simulink model "Thesis_MMC_WF_Modify"  (R2023a)
settings: Solver=VariableStepAuto  StartTime=0.0  StopTime=16  RelTol=1e-3
InitFcn:
  | % TS %
  | Ts_Control=4e-05;
  | Ts_Power=2e-05;
  | %% Main Circuit %%
  | % AC Line %
  | Vnom_Sec=333000;
  | Vnom_Pri=400000;
  | Pnom=1.0e+09;
  | Fnom=60;
  | Psc=2.0e+10;
  | P_Ld1=2/3*1e+09;
  | R_Startup=400;
  | Rxfo=0.003;
  | Lxfo=0.12;
  | P_Ld2=500e+03;
  | % MMC Parameter %
  | Larm_pu=0.15;
  | Rarm_pu=Larm_pu/100;
  | Zbase= Vnom_Sec^2/Pnom;
  | Larm=Larm_pu*(Zbase/(2*pi*Fnom));
  | Rarm=Rarm_pu*Zbase;
  | C_PM=1.758e-3;
  | w=2*pi*Fnom;
  | wc2=(2*w)^2;
  | Cfilter=1/(Larm*wc2);
  | Rfilter=1/(Cfilter*w)*30;
  | Topen_Filter=1e6;
  | K_V_dc=600000;
  | n=36;
  | Rg=100;
  | Cg=5e-08;
  | % HVDC Parameter %
  | R_cable=0.5;
  | L_cable=0.015;
  | %% Controller Parameter %%
  | % PLL %
  | Fn_filter=1000;
  | Zeta_filter=1;
  | % Active Power Regulator %
  | Kp_Preg=1/6;
  | Ki_Preg=1;
  | Limits_Preg=[0.8 1.2];
  | set_param('Thesis_MMC_WF_Modify/Controller/Active Power Regulator/Sum1','SampleTime','Ts_Control')
  | set_param('Thesis_MMC_WF_Modify/Controller/Active Power Regulator/Saturation','SampleTime','Ts_Control')
  | % Reactive Power Regulator %
  | Kp_Qreg=1/6;
  | Ki_Qreg=1;
  | Limits_Qreg=[-0.25 0.25];
  | set_param('Thesis_MMC_WF_Modify/Controller/Reactive Power Regulartor/Sum1','SampleTime','Ts_Control')
  | % Discrete Mean %
  | K1=3.2312e-30;
  | K2=-1.1369e-16;
  | Delay=0.02;
  | Vint=0;
  | Delay1=0.02004;
  | % DC Voltage Regulator %
  | Kp_VDCreg=4;
  | Ki_VDCreg=100;
  | Limits_VDCreg=[-2 2];
  | set_param('Thesis_MMC_WF_Modify/Controller/DC Voltage Regulator/Sum1','SampleTime','Ts_Control')
  | set_param('Thesis_MMC_WF_Modify/Controller/DC Voltage Regulator/Saturation','SampleTime','Ts_Control')
  | % Current Regulator %
  | Limits_Ireg=[-2 2];
  | Lff=0.075;
  | Rff=0.00075;
  | % PI Regulator %
  | Kp=0.6;
  | Ki=6;
  | UpperLimit=2;
  | LowerLimit=-2;
  | set_param('Thesis_MMC_WF_Modify/Controller/Current Regular/PI Regulator1/Sum1','SampleTime','Ts_Control')
  | set_param('Thesis_MMC_WF_Modify/Controller/Current Regular/PI Regulator1/Sum2','SampleTime','Ts_Control')
  | set_param('Thesis_MMC_WF_Modify/Controller/Current Regular/PI Regulator1/Gain1','SampleTime','Ts_Control')
  | set_param('Thesis_MMC_WF_Modify/Controller/Current Regular/PI Regulator1/Gain2','SampleTime','Ts_Control')
  | set_param('Thesis_MMC_WF_Modify/Controller/Current Regular/PI Regulator1/Saturation','SampleTime','Ts_Control')
  | set_param('Thesis_MMC_WF_Modify/Controller/Current Regular/PI Regulator2/Sum1','SampleTime','Ts_Control')
  | set_param('Thesis_MMC_WF_Modify/Controller/Current Regular/PI Regulator2/Sum2','SampleTime','Ts_Control')
  | set_param('Thesis_MMC_WF_Modify/Controller/Current Regular/PI Regulator2/Gain1','SampleTime','Ts_Control')
  | set_param('Thesis_MMC_WF_Modify/Controller/Current Regular/PI Regulator2/Gain2','SampleTime','Ts_Control')
  | set_param('Thesis_MMC_WF_Modify/Controller/Current Regular/PI Regulator2/Saturation','SampleTime','Ts_Control')
  | % PWM Generator %
  | pp=0;
  | for p=1:2:72
  | pp=pp+1;
  | SelectPulses1(p)=pp;
  | SelectPulses1(p+1)=pp+36;
  | end
  | Offse_Cr=0:0.000137377733816902958333333:35*0.000137377733816902958333333;
  | Fc=Fnom*3.37;
  | Tc=0.004945598417408506583333333;
  | %% Sequence & Slope %%
  | TBrk1_On=0.1;
  | TBrk2_On=1;
  | Ton_VDCreg=1.5;
  | Slope_Vdc_ref=128000;
  | Tramping_Vdc_ref=2;
  | Slope_Pref=0.5;
  | Ton_PQreg=4;
  | Tramping_Pref=4.2;
  | Slope_Qref=0.5;
  | Tramping_Qref=7.0;
  | Limits_Qreg=[-0.25 0.25];
  | %% Fault Time %%
  | T_Fault=10;
  | %% 12-Pulse %%
  | R_12_arm=0.001;
undefined symbols (not defined in the file): D1, Delta, Delta1, DiscIntNeverNeededParam, Lagging, Vnom_dc
libraries: spsSeriesRLCBranchLib x54, spsIGBTLib x24, spsBreakerLib x13, spsVoltageMeasurementLib x11, spsThreePhaseBreakerLib x11, spsThreePhaseVIMeasurementLib x9, spsIdealSwitchLib x8, simulink x7, spsDiscreteVariableTimeDelayLib x7, spsCurrentMeasurementLib x6, spsGroundLib x6, spsSecondOrderFilterLib x6
(part 1 of 3)
settings Model: SimulationMode=accelerator  Creator=GW Smart Grid Lab  LastModifiedBy=hwang22
settings OptimizationCC: ReuseModelBlockBuffer=off

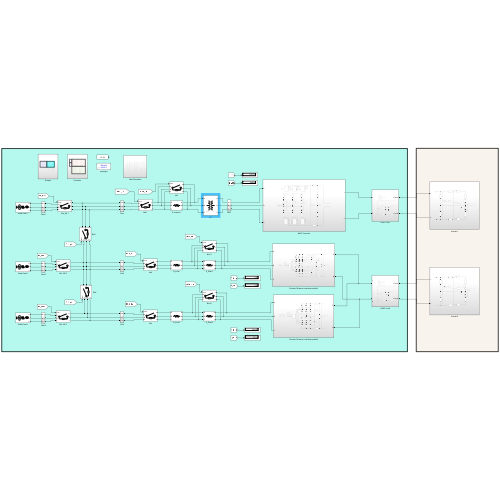
[thumbnail: Simulink's stored preview of the top-level diagram]
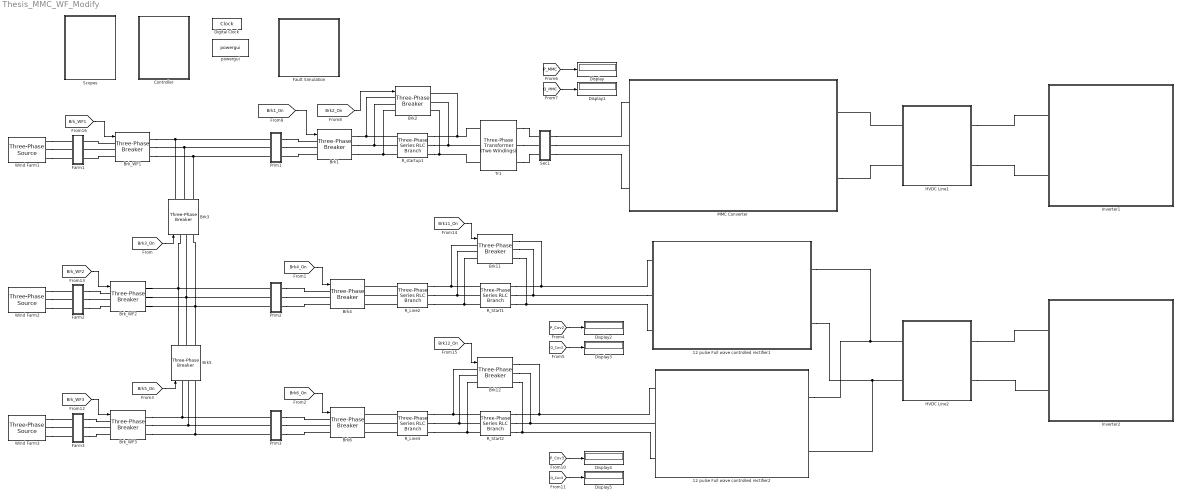
== system Thesis_MMC_WF_Modify ==
  12 pulse Full wave controlled rectifier1 : Subsystem
  12 pulse Full wave controlled rectifier2 : Subsystem
  Brk1 : spsThreePhaseBreakerLib/Three-Phase Breaker  InitialState=open  SwitchA=on  SwitchB=on  SwitchC=on  SwitchTimes=0.1  External=on  BreakerResistance=0.001  SnubberResistance=1e6  SnubberCapacitance=inf  Measurements=None
  Brk{3..6,11..12} (6 alike) : spsThreePhaseBreakerLib/Three-Phase Breaker  InitialState=open  SwitchA=on  SwitchB=on  SwitchC=on  SwitchTimes="[1/60  5/60]"  External=on  BreakerResistance=0.01  SnubberResistance=1e6  SnubberCapacitance=inf  Measurements=None
  Brk2 : spsThreePhaseBreakerLib/Three-Phase Breaker  InitialState=open  SwitchA=on  SwitchB=on  SwitchC=on  SwitchTimes=[30/60]*10000  External=on  BreakerResistance=0.01  SnubberResistance=1e6  SnubberCapacitance=inf  Measurements=None
  Brk_WF1 : spsThreePhaseBreakerLib/Three-Phase Breaker  InitialState=open  SwitchA=on  SwitchB=on  SwitchC=on  SwitchTimes="[1/60  5/60]"  External=on  BreakerResistance=0.01  SnubberResistance=1e6  SnubberCapacitance=inf  Measurements=None
  Brk_WF2 : spsThreePhaseBreakerLib/Three-Phase Breaker  InitialState=open  SwitchA=on  SwitchB=on  SwitchC=on  SwitchTimes="[1/60  5/60]"  External=on  BreakerResistance=0.01  SnubberResistance=1e6  SnubberCapacitance=inf  Measurements=None
  Brk_WF3 : spsThreePhaseBreakerLib/Three-Phase Breaker  InitialState=open  SwitchA=on  SwitchB=on  SwitchC=on  SwitchTimes="[1/60  5/60]"  External=on  BreakerResistance=0.01  SnubberResistance=1e6  SnubberCapacitance=inf  Measurements=None
  Controller : Subsystem
  Digital Clock : DigitalClock  SampleTime=Ts_Control
  Display{,1..5} (6 alike) : Display
      settings: Format=bank  Decimation=500
  Farm1 : Subsystem
  Farm2 : Subsystem
  Farm3 : Subsystem
  Fault Simulation : Subsystem
  HVDC Line1 : Subsystem
  HVDC Line2 : Subsystem
  Inverter1 : Subsystem
  Inverter2 : Subsystem
  MMC Converter : Subsystem
  Prim1 : Subsystem
  Prim2 : Subsystem
  Prim3 : Subsystem
  R_Line2 : spsThreePhaseSeriesRLCBranchLib/Three-Phase Series RLC Branch  LConnTagsString=A|B|C  RConnTagsString=A|B|C  BranchType=R  Resistance=10*0.007  Inductance=1e-3  Capacitance=1e-6  Measurements=None
  R_Line3 : spsThreePhaseSeriesRLCBranchLib/Three-Phase Series RLC Branch  LConnTagsString=A|B|C  RConnTagsString=A|B|C  BranchType=R  Resistance=10*0.007  Inductance=1e-3  Capacitance=1e-6  Measurements=None
  R_Start1 : spsThreePhaseSeriesRLCBranchLib/Three-Phase Series RLC Branch  LConnTagsString=A|B|C  RConnTagsString=A|B|C  BranchType=R  Resistance=540*0.01  Inductance=1e-3  Capacitance=1e-6  Measurements=None
  R_Start2 : spsThreePhaseSeriesRLCBranchLib/Three-Phase Series RLC Branch  LConnTagsString=A|B|C  RConnTagsString=A|B|C  BranchType=R  Resistance=540*0.01  Inductance=1e-3  Capacitance=1e-6  Measurements=None
  R_startup1 : spsThreePhaseSeriesRLCBranchLib/Three-Phase Series RLC Branch  LConnTagsString=A|B|C  RConnTagsString=A|B|C  BranchType=R  Resistance=R_Startup/100  Inductance=1e-3  Capacitance=1e-6  Measurements=None
  Scopes : Subsystem
  Sec1 : Subsystem
  Tr1 : spsThreePhaseTransformerTwoWindingsLib/Three-Phase Transformer (Two Windings)  Winding1Connection=Yg  Winding2Connection=Y  CoreType=Three single-phase transformers  SetSaturation=off  Hysteresis=off  DataFile='hysteresis'  SetInitialFlux=off  Measurements=None  UNITS=pu  NominalPower=[ Pnom , Fnom ]  Winding1="[ Vnom_Pri*0.1 , Rxfo/2,  Lxfo/2 ]"  Winding2="[ Vnom_Sec , Rxfo/2,  Lxfo/2 ]"  Rm=1000  Lm=1000  L0=0.5  Saturation=[ 0,0 ; 0.0024,1.2 ; 1.0,1.52 ]  InitialFluxes=[ 0.8 , -0.8 , 0.7 ]  BreakLoop=off  DiscreteSolver=Trapezoidal iterative  DataType=off  TransfoNumber=1
  Wind Farm1 : spsThreePhaseSourceLib/Three-Phase Source  InternalConnection=Yg  VoltagePhases=off  Voltage=Vnom_Pri*0.099  PhaseAngle=0  Voltage_phases=[25e3 25e3 25e3]/sqrt(3)  PhaseAngles_phases=[0 -120 +120]  Frequency=Fnom  NonIdealSource=on  SpecifyImpedance=on  Resistance=0.8929  Inductance=16.58e-3  ShortCircuitLevel=Psc  BaseVoltage=Vnom_Pri*0.1  XRratio=7  BusType=PQ  Pref=1.0e9  Qref=2.5e8  Prefabc=[10e3, 10e3, 10e3]  Qrefabc=[0, 0, 0]  Qmin=-inf  Qmax=inf
  Wind Farm2 : spsThreePhaseSourceLib/Three-Phase Source  InternalConnection=Yg  VoltagePhases=off  Voltage=Vnom_Pri*0.099  PhaseAngle=0  Voltage_phases=[25e3 25e3 25e3]/sqrt(3)  PhaseAngles_phases=[0 -120 +120]  Frequency=Fnom  NonIdealSource=on  SpecifyImpedance=on  Resistance=0.8929  Inductance=16.58e-3  ShortCircuitLevel=Psc  BaseVoltage=Vnom_Pri*0.1  XRratio=7  BusType=PQ  Pref=1.2e9  Qref=2.5e8  Prefabc=[10e3, 10e3, 10e3]  Qrefabc=[0, 0, 0]  Qmin=-inf  Qmax=inf
  Wind Farm3 : spsThreePhaseSourceLib/Three-Phase Source  InternalConnection=Yg  VoltagePhases=off  Voltage=Vnom_Pri*0.099  PhaseAngle=0  Voltage_phases=[25e3 25e3 25e3]/sqrt(3)  PhaseAngles_phases=[0 -120 +120]  Frequency=Fnom  NonIdealSource=on  SpecifyImpedance=on  Resistance=0.8929  Inductance=16.58e-3  ShortCircuitLevel=Psc  BaseVoltage=Vnom_Pri*0.1  XRratio=7  BusType=PQ  Pref=1.0e9  Qref=2.5e8  Prefabc=[10e3, 10e3, 10e3]  Qrefabc=[0, 0, 0]  Qmin=-inf  Qmax=inf
  powergui : spspowerguiLib/powergui  Priority=1  SimulationMode=Discrete  SampleTime=Ts_Power  frequency=60  Iterations=50  frequencyindice=60  Pbase=100e6  ErrMax=1e-4  UnitsV=kV  UnitsW=MW  buscounter=0  FunctionMessages=off  echomessages=off  EnableUseOfTLC=off  CurrentSourceSwitches=off  DisableSnubberDevices=off  DisableRonSwitches=off  DisableVfSwitches=off  DisplayEquations=off  AutomaticDiscreteSolvers=off  SolverType=Tustin/Backward Euler (TBE)  Interpol=off  ExternalGateDelay=off  methode=off  Ts=100  x0status=blocks  SPID=on  SwTol=0  HookPort=off  NonlinearTolerance=1e-4  nMaxIteration=100  ContinueOnMaxIteration=off  RestoreLinks=warning  ResistiveCurrentMeasurement=off  Frange=[0:2:500]  Ylog=off  Xlog=on  ShowGrid=off  save=off  variable=ZData  structure=0  ZoomFFT=off  StartTime=0.0  cycles=1  DisplayStyle=1  fundamental=60  FreqAxis=off  MaxFrequency=1000  frequencyindicesteady=1  RmsSteady=1  display=off
  wires:
  [Brk2_On] -> Brk2/1
  [Brk1_On] -> Brk1/1
  [Brk3_On] -> Brk3/1
  [Brk4_On] -> Brk4/1
  [Brk6_On] -> Brk6/1
  [Brk5_On] -> Brk5/1
  [P_MMC] -> Display/1
  [Q_MMC] -> Display1/1
  [Brk11_On] -> Brk11/1
  [Brk12_On] -> Brk12/1
  [Q_Cov2] -> Display3/1
  [P_Cov2] -> Display2/1
  [P_Cov3] -> Display4/1
  [Q_Cov3] -> Display5/1
  [Brk_WF3] -> Brk_WF3/1
  [Brk_WF2] -> Brk_WF2/1
  [Brk_WF1] -> Brk_WF1/1
  connections:
  R_startup1/RConn1 -- Tr1/LConn1 -- Brk2/RConn1
  Tr1/RConn3 -- Sec1/LConn3
  Tr1/RConn2 -- Sec1/LConn2
  Brk2/LConn1 -- Brk1/RConn1 -- R_startup1/LConn1
  Brk2/LConn2 -- Brk1/RConn2 -- R_startup1/LConn2
  Brk2/LConn3 -- Brk1/RConn3 -- R_startup1/LConn3
  Tr1/RConn1 -- Sec1/LConn1
  R_startup1/RConn2 -- Tr1/LConn2 -- Brk2/RConn2
  R_startup1/RConn3 -- Tr1/LConn3 -- Brk2/RConn3
  HVDC Line1/RConn1 -- Inverter1/LConn1
  HVDC Line1/RConn2 -- Inverter1/LConn2
  Brk1/LConn3 -- Prim1/RConn3
  Prim1/RConn2 -- Brk1/LConn2
  Prim1/RConn1 -- Brk1/LConn1
  Sec1/RConn1 -- MMC Converter/LConn1
  Sec1/RConn2 -- MMC Converter/LConn2
  Sec1/RConn3 -- MMC Converter/LConn3
  Brk5/RConn2 -- Brk_WF2/RConn2 -- Prim2/LConn2 -- Brk3/LConn2
  Brk5/RConn1 -- Brk_WF2/RConn1 -- Brk3/LConn1 -- Prim2/LConn1
  12 pulse Full wave controlled rectifier1/LConn1 -- R_Start1/RConn1 -- Brk11/RConn1
  12 pulse Full wave controlled rectifier1/LConn2 -- R_Start1/RConn2 -- Brk11/RConn2
  12 pulse Full wave controlled rectifier1/LConn3 -- R_Start1/RConn3 -- Brk11/RConn3
  HVDC Line1/LConn1 -- MMC Converter/RConn1
  MMC Converter/RConn2 -- HVDC Line1/LConn2
  12 pulse Full wave controlled rectifier2/LConn1 -- Brk12/RConn1 -- R_Start2/RConn1
  R_Start2/LConn2 -- R_Line3/RConn2 -- Brk12/LConn2
  R_Start2/LConn3 -- R_Line3/RConn3 -- Brk12/LConn3
  12 pulse Full wave controlled rectifier1/RConn1 -- 12 pulse Full wave controlled rectifier2/RConn1 -- HVDC Line2/LConn1
  Prim2/RConn3 -- Brk4/LConn3
  Prim2/RConn2 -- Brk4/LConn2
  Prim2/RConn1 -- Brk4/LConn1
  Prim3/RConn1 -- Brk6/LConn1
  Prim3/RConn2 -- Brk6/LConn2
  Prim3/RConn3 -- Brk6/LConn3
  HVDC Line2/RConn1 -- Inverter2/LConn1
  HVDC Line2/RConn2 -- Inverter2/LConn2
  Prim3/LConn1 -- Brk5/LConn1 -- Brk_WF3/RConn1
  HVDC Line2/LConn2 -- 12 pulse Full wave controlled rectifier1/RConn2 -- 12 pulse Full wave controlled rectifier2/RConn2
  Wind Farm1/RConn1 -- Farm1/LConn1
  Wind Farm1/RConn2 -- Farm1/LConn2
  Wind Farm1/RConn3 -- Farm1/LConn3
  R_Start1/LConn1 -- R_Line2/RConn1 -- Brk11/LConn1
  R_Start1/LConn2 -- R_Line2/RConn2 -- Brk11/LConn2
  R_Start1/LConn3 -- R_Line2/RConn3 -- Brk11/LConn3
  Brk12/RConn3 -- R_Start2/RConn3 -- 12 pulse Full wave controlled rectifier2/LConn3
  R_Start2/LConn1 -- R_Line3/RConn1 -- Brk12/LConn1
  Brk12/RConn2 -- R_Start2/RConn2 -- 12 pulse Full wave controlled rectifier2/LConn2
  Wind Farm2/RConn1 -- Farm2/LConn1
  Wind Farm2/RConn2 -- Farm2/LConn2
  Wind Farm2/RConn3 -- Farm2/LConn3
  Wind Farm3/RConn1 -- Farm3/LConn1
  Wind Farm3/RConn2 -- Farm3/LConn2
  Wind Farm3/RConn3 -- Farm3/LConn3
  Prim3/LConn3 -- Brk_WF3/RConn3 -- Brk5/LConn3
  Prim3/LConn2 -- Brk_WF3/RConn2 -- Brk5/LConn2
  Brk5/RConn3 -- Brk_WF2/RConn3 -- Prim2/LConn3 -- Brk3/LConn3
  Brk_WF1/RConn1 -- Brk3/RConn1 -- Prim1/LConn1
  Brk_WF1/RConn2 -- Brk3/RConn2 -- Prim1/LConn2
  Brk_WF1/RConn3 -- Brk3/RConn3 -- Prim1/LConn3
  Brk_WF1/LConn1 -- Farm1/RConn1
  Brk_WF1/LConn2 -- Farm1/RConn2
  Brk_WF1/LConn3 -- Farm1/RConn3
  Farm2/RConn3 -- Brk_WF2/LConn3
  Farm2/RConn2 -- Brk_WF2/LConn2
  Farm2/RConn1 -- Brk_WF2/LConn1
  Farm3/RConn3 -- Brk_WF3/LConn3
  Farm3/RConn2 -- Brk_WF3/LConn2
  Farm3/RConn1 -- Brk_WF3/LConn1
  R_Line2/LConn1 -- Brk4/RConn1
  R_Line2/LConn2 -- Brk4/RConn2
  R_Line2/LConn3 -- Brk4/RConn3
  R_Line3/LConn2 -- Brk6/RConn2
  R_Line3/LConn3 -- Brk6/RConn3
  R_Line3/LConn1 -- Brk6/RConn1

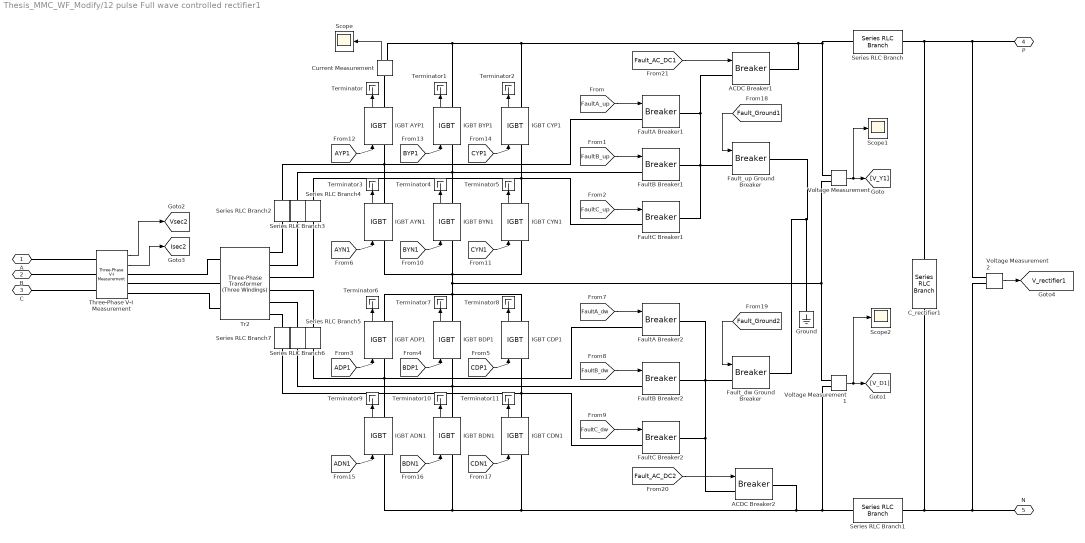
== system Thesis_MMC_WF_Modify/12 pulse Full wave controlled rectifier1 ==
  ACDC Breaker1 : spsBreakerLib/Breaker  InitialState=0  SwitchingTimes="[1/60  5/60]"  External=on  BreakerResistance=0.01  SnubberResistance=1e6  SnubberCapacitance=inf  Measurements=None  MoreParameters=on  NoBreakLoop=off
  ACDC Breaker2 : spsBreakerLib/Breaker  InitialState=0  SwitchingTimes="[1/60  5/60]"  External=on  BreakerResistance=0.01  SnubberResistance=1e6  SnubberCapacitance=inf  Measurements=None  MoreParameters=on  NoBreakLoop=off
  C_rectifier1 : spsSeriesRLCBranchLib/Series RLC Branch  LConnTagsString=__new0  RConnTagsString=__new0  BranchType=C  Resistance=1  Inductance=1e-3  SetiL0=off  InitialCurrent=0  Capacitance=5e-4  Setx0=off  InitialVoltage=0  Measurements=None
  Current Measurement : spsCurrentMeasurementLib/Current Measurement  PhasorSimulation=off  OutputType=Complex  PSBequivalent=0
  FaultA Breaker1 : spsBreakerLib/Breaker  InitialState=0  SwitchingTimes="[1/60  5/60]"  External=on  BreakerResistance=0.01  SnubberResistance=1e6  SnubberCapacitance=inf  Measurements=None  MoreParameters=on  NoBreakLoop=off
  FaultA Breaker2 : spsBreakerLib/Breaker  InitialState=0  SwitchingTimes="[1/60  5/60]"  External=on  BreakerResistance=0.01  SnubberResistance=1e6  SnubberCapacitance=inf  Measurements=None  MoreParameters=on  NoBreakLoop=off
  FaultB Breaker1 : spsBreakerLib/Breaker  InitialState=0  SwitchingTimes="[1/60  5/60]"  External=on  BreakerResistance=0.01  SnubberResistance=1e6  SnubberCapacitance=inf  Measurements=None  MoreParameters=on  NoBreakLoop=off
  FaultB Breaker2 : spsBreakerLib/Breaker  InitialState=0  SwitchingTimes="[1/60  5/60]"  External=on  BreakerResistance=0.01  SnubberResistance=1e6  SnubberCapacitance=inf  Measurements=None  MoreParameters=on  NoBreakLoop=off
  FaultC Breaker1 : spsBreakerLib/Breaker  InitialState=0  SwitchingTimes="[1/60  5/60]"  External=on  BreakerResistance=0.01  SnubberResistance=1e6  SnubberCapacitance=inf  Measurements=None  MoreParameters=on  NoBreakLoop=off
  FaultC Breaker2 : spsBreakerLib/Breaker  InitialState=0  SwitchingTimes="[1/60  5/60]"  External=on  BreakerResistance=0.01  SnubberResistance=1e6  SnubberCapacitance=inf  Measurements=None  MoreParameters=on  NoBreakLoop=off
  Fault_dw Ground Breaker : spsBreakerLib/Breaker  InitialState=0  SwitchingTimes="[1/60  5/60]"  External=on  BreakerResistance=0.01  SnubberResistance=1e6  SnubberCapacitance=inf  Measurements=None  MoreParameters=on  NoBreakLoop=off
  Fault_up Ground Breaker : spsBreakerLib/Breaker  InitialState=0  SwitchingTimes="[1/60  5/60]"  External=on  BreakerResistance=0.01  SnubberResistance=1e6  SnubberCapacitance=inf  Measurements=None  MoreParameters=on  NoBreakLoop=off
  Ground : spsGroundLib/Ground  LConnTagsString=a
  IGBT ADN1 : spsIGBTLib/IGBT  Ron=0.001  Lon=0  Vf=1  Tf=1e-6  Tt=2e-6  IC=0  Rs=1e5  Cs=inf  Measurements=on
  IGBT ADP1 : spsIGBTLib/IGBT  Ron=0.001  Lon=0  Vf=1  Tf=1e-6  Tt=2e-6  IC=0  Rs=1e5  Cs=inf  Measurements=on
  IGBT AYN1 : spsIGBTLib/IGBT  Ron=0.001  Lon=0  Vf=1  Tf=1e-6  Tt=2e-6  IC=0  Rs=1e5  Cs=inf  Measurements=on
  IGBT AYP1 : spsIGBTLib/IGBT  Ron=0.001  Lon=0  Vf=1  Tf=1e-6  Tt=2e-6  IC=0  Rs=1e5  Cs=inf  Measurements=on
  IGBT BDN1 : spsIGBTLib/IGBT  Ron=0.001  Lon=0  Vf=1  Tf=1e-6  Tt=2e-6  IC=0  Rs=1e5  Cs=inf  Measurements=on
  IGBT BDP1 : spsIGBTLib/IGBT  Ron=0.001  Lon=0  Vf=1  Tf=1e-6  Tt=2e-6  IC=0  Rs=1e5  Cs=inf  Measurements=on
  IGBT BYN1 : spsIGBTLib/IGBT  Ron=0.001  Lon=0  Vf=1  Tf=1e-6  Tt=2e-6  IC=0  Rs=1e5  Cs=inf  Measurements=on
  IGBT BYP1 : spsIGBTLib/IGBT  Ron=0.001  Lon=0  Vf=1  Tf=1e-6  Tt=2e-6  IC=0  Rs=1e5  Cs=inf  Measurements=on
  IGBT CDN1 : spsIGBTLib/IGBT  Ron=0.001  Lon=0  Vf=1  Tf=1e-6  Tt=2e-6  IC=0  Rs=1e5  Cs=inf  Measurements=on
  IGBT CDP1 : spsIGBTLib/IGBT  Ron=0.001  Lon=0  Vf=1  Tf=1e-6  Tt=2e-6  IC=0  Rs=1e5  Cs=inf  Measurements=on
  IGBT CYN1 : spsIGBTLib/IGBT  Ron=0.001  Lon=0  Vf=1  Tf=1e-6  Tt=2e-6  IC=0  Rs=1e5  Cs=inf  Measurements=on
  IGBT CYP1 : spsIGBTLib/IGBT  Ron=0.001  Lon=0  Vf=1  Tf=1e-6  Tt=2e-6  IC=0  Rs=1e5  Cs=inf  Measurements=on
  Scope : Scope
  Scope1 : Scope
  Scope2 : Scope
  Series RLC Branch : spsSeriesRLCBranchLib/Series RLC Branch  LConnTagsString=__new0  RConnTagsString=__new0  BranchType=L  Resistance=1  Inductance=0.0004  SetiL0=off  InitialCurrent=0  Capacitance=1e-6  Setx0=off  InitialVoltage=0  Measurements=None
  Series RLC Branch1 : spsSeriesRLCBranchLib/Series RLC Branch  LConnTagsString=__new0  RConnTagsString=__new0  BranchType=L  Resistance=1  Inductance=0.0004  SetiL0=off  InitialCurrent=0  Capacitance=1e-6  Setx0=off  InitialVoltage=0  Measurements=None
  Series RLC Branch{2..7} (6 alike) : spsSeriesRLCBranchLib/Series RLC Branch  LConnTagsString=__new0  RConnTagsString=__new0  BranchType=RL  Resistance=R_12_arm  Inductance=1e-3  SetiL0=off  InitialCurrent=0  Capacitance=1e-6  Setx0=off  InitialVoltage=0  Measurements=None
  Terminator{,1..11} (12 alike) : Terminator
  Three-Phase V-I Measurement : spsThreePhaseVIMeasurementLib/Three-Phase V-I Measurement  VoltageMeasurement=phase-to-ground  SetLabelV=off  LabelV=Vabc  Vpu=off  VpuLL=off  CurrentMeasurement=yes  SetLabelI=off  LabelI=Iabc  Ipu=off  Pbase=100e6  Vbase=500e3  OutputType=Complex  PhasorSimulation=off  PSBequivalent=0
  Tr2 : spsThreePhaseTransformerThreeWindingsLib/Three-Phase Transformer (Three Windings)  Winding1Connection=Yg  Winding2Connection=Y  Winding3Connection=Delta (D1)  CoreType=Three single-phase transformers  SetSaturation=off  Hysteresis=off  DataFile='hysteresis'  SetInitialFlux=off  Measurements=None  UNITS=pu  NominalPower=[ 2.5e9 , 60 ]  Winding1=[ 4e+5*0.1 , 0.002 , 0.08 ]  Winding2=[ 2.675e+5 , 0.002 , 0.08 ]  Winding3=[2.675e+5 , 0.002 , 0.08 ]  Rm=1000  Lm=1000  L0=0.5  Saturation=[ 0,0 ; 0.0024,1.2 ; 1.0,1.52 ]  InitialFluxes=[0.8 -0.8 0.7]  BreakLoop=off  DiscreteSolver=Trapezoidal iterative  DataType=off  TransfoNumber=1
      settings: LibrarySourceBlock=|
      | sps_lib/Power Grid Elements/Three-Phase
      | Transformer
      | (Three Windings)
  Voltage Measurement : spsVoltageMeasurementLib/Voltage Measurement  PhasorSimulation=off  OutputType=Complex  PSBequivalent=0
  Voltage Measurement1 : spsVoltageMeasurementLib/Voltage Measurement  PhasorSimulation=off  OutputType=Complex  PSBequivalent=0
  Voltage Measurement2 : spsVoltageMeasurementLib/Voltage Measurement  PhasorSimulation=off  OutputType=Complex  PSBequivalent=0
  A : PMIOPort  Side=Left
  B : PMIOPort  Port=2  Side=Left
  C : PMIOPort  Port=3  Side=Left
  P : PMIOPort  Port=4  Side=Right
  N : PMIOPort  Port=5  Side=Right
  tag scope: Isec2=global, V_rectifier1=global, Vsec2=global
  wires:
  IGBT BDN1/1 -> Terminator10/1
  IGBT CYP1/1 -> Terminator2/1
  IGBT BDP1/1 -> Terminator7/1
  IGBT AYN1/1 -> Terminator3/1
  IGBT BYP1/1 -> Terminator1/1
  [BYN1] -> IGBT BYN1/1
  IGBT CDN1/1 -> Terminator11/1
  [CYP1] -> IGBT CYP1/1
  IGBT CYN1/1 -> Terminator5/1
  IGBT AYP1/1 -> Terminator/1
  [BDN1] -> IGBT BDN1/1
  [BDP1] -> IGBT BDP1/1
  [CDN1] -> IGBT CDN1/1
  [BYP1] -> IGBT BYP1/1
  [CDP1] -> IGBT CDP1/1
  IGBT CDP1/1 -> Terminator8/1
  IGBT BYN1/1 -> Terminator4/1
  [ADP1] -> IGBT ADP1/1
  [ADN1] -> IGBT ADN1/1
  [AYN1] -> IGBT AYN1/1
  [CYN1] -> IGBT CYN1/1
  IGBT ADP1/1 -> Terminator6/1
  IGBT ADN1/1 -> Terminator9/1
  Voltage Measurement/1 -> Scope1/1, [V_Y1]
  Voltage Measurement1/1 -> Scope2/1, [V_D1]
  Three-Phase V-I Measurement/1 -> [Vsec2]
  Three-Phase V-I Measurement/2 -> [Isec2]
  Voltage Measurement2/1 -> [V_rectifier1]
  [FaultA_up] -> FaultA Breaker1/1
  [FaultB_up] -> FaultB Breaker1/1
  [FaultC_up] -> FaultC Breaker1/1
  [FaultA_dw] -> FaultA Breaker2/1
  [FaultB_dw] -> FaultB Breaker2/1
  [FaultC_dw] -> FaultC Breaker2/1
  [Fault_Ground1] -> Fault_up Ground Breaker/1
  [Fault_Ground2] -> Fault_dw Ground Breaker/1
  [Fault_AC_DC2] -> ACDC Breaker2/1
  [Fault_AC_DC1] -> ACDC Breaker1/1
  Current Measurement/1 -> Scope/1
  [AYP1] -> IGBT AYP1/1
  connections:
  IGBT ADN1/RConn1 -- Series RLC Branch5/RConn1 -- FaultA Breaker2/LConn1 -- IGBT ADP1/LConn1
  Voltage Measurement/LConn1 -- Series RLC Branch/LConn1 -- ACDC Breaker1/RConn1 -- IGBT CYP1/RConn1 -- Current Measurement/RConn1 -- IGBT BYP1/RConn1
  FaultA Breaker1/LConn1 -- Series RLC Branch2/LConn1 -- IGBT AYN1/RConn1 -- IGBT AYP1/LConn1
  IGBT CDP1/RConn1 -- Voltage Measurement1/LConn1 -- Voltage Measurement/LConn2 -- IGBT CYN1/LConn1 -- IGBT BYN1/LConn1 -- IGBT AYN1/LConn1 -- IGBT BDP1/RConn1 -- IGBT ADP1/RConn1
  IGBT CYN1/RConn1 -- Series RLC Branch4/LConn1 -- FaultC Breaker1/LConn1 -- IGBT CYP1/LConn1
  FaultA Breaker2/RConn1 -- FaultC Breaker2/RConn1 -- ACDC Breaker2/LConn1 -- Fault_dw Ground Breaker/LConn1 -- FaultB Breaker2/RConn1
  FaultB Breaker1/LConn1 -- IGBT BYP1/LConn1 -- Series RLC Branch3/LConn1 -- IGBT BYN1/RConn1
  IGBT CDN1/RConn1 -- Series RLC Branch7/RConn1 -- FaultC Breaker2/LConn1 -- IGBT CDP1/LConn1
  IGBT BDN1/RConn1 -- Series RLC Branch6/RConn1 -- IGBT BDP1/LConn1 -- FaultB Breaker2/LConn1
  Three-Phase V-I Measurement/RConn1 -- Tr2/LConn1
  Three-Phase V-I Measurement/RConn3 -- Tr2/LConn3
  Three-Phase V-I Measurement/RConn2 -- Tr2/LConn2
  A/RConn1 -- Three-Phase V-I Measurement/LConn1
  B/RConn1 -- Three-Phase V-I Measurement/LConn2
  C/RConn1 -- Three-Phase V-I Measurement/LConn3
  Voltage Measurement2/LConn1 -- C_rectifier1/LConn1 -- Series RLC Branch/RConn1 -- P/RConn1
  Voltage Measurement2/LConn2 -- Series RLC Branch1/RConn1 -- C_rectifier1/RConn1 -- N/RConn1
  Fault_up Ground Breaker/RConn1 -- Fault_dw Ground Breaker/RConn1 -- Ground/LConn1
  Voltage Measurement1/LConn2 -- Series RLC Branch1/LConn1 -- ACDC Breaker2/RConn1 -- IGBT CDN1/LConn1 -- IGBT BDN1/LConn1 -- IGBT ADN1/LConn1
  FaultA Breaker1/RConn1 -- Fault_up Ground Breaker/LConn1 -- FaultC Breaker1/RConn1 -- FaultB Breaker1/RConn1 -- ACDC Breaker1/LConn1
  Tr2/RConn1 -- Series RLC Branch2/RConn1
  Tr2/RConn2 -- Series RLC Branch3/RConn1
  Tr2/RConn3 -- Series RLC Branch4/RConn1
  Tr2/RConn4 -- Series RLC Branch5/LConn1
  Tr2/RConn5 -- Series RLC Branch6/LConn1
  Tr2/RConn6 -- Series RLC Branch7/LConn1
  IGBT AYP1/RConn1 -- Current Measurement/LConn1

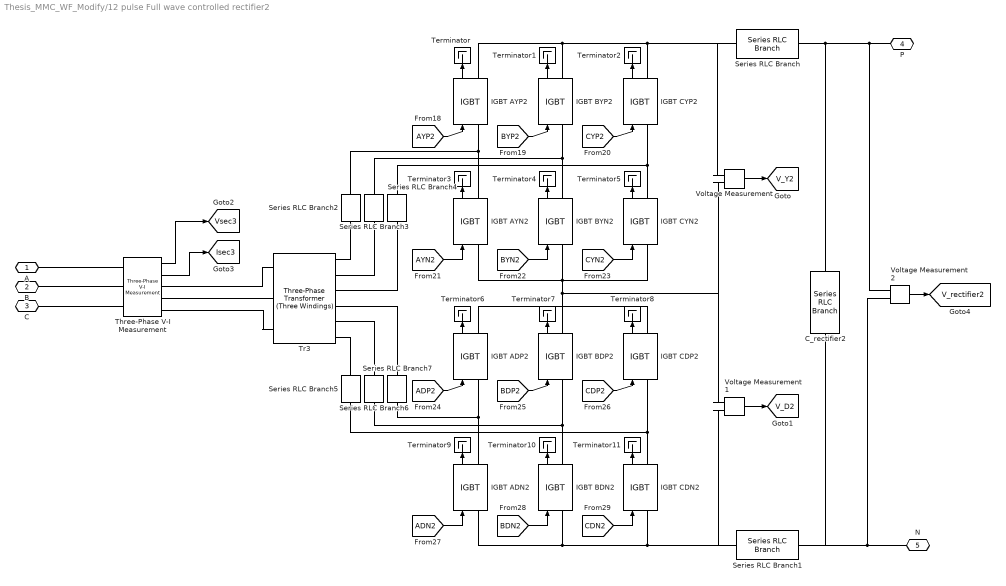
== system Thesis_MMC_WF_Modify/12 pulse Full wave controlled rectifier2 ==
  C_rectifier2 : spsSeriesRLCBranchLib/Series RLC Branch  LConnTagsString=__new0  RConnTagsString=__new0  BranchType=C  Resistance=1  Inductance=1e-3  SetiL0=off  InitialCurrent=0  Capacitance=5e-4  Setx0=off  InitialVoltage=0  Measurements=None
  IGBT ADN2 : spsIGBTLib/IGBT  Ron=0.001  Lon=0  Vf=1  Tf=1e-6  Tt=2e-6  IC=0  Rs=1e5  Cs=inf  Measurements=on
  IGBT ADP2 : spsIGBTLib/IGBT  Ron=0.001  Lon=0  Vf=1  Tf=1e-6  Tt=2e-6  IC=0  Rs=1e5  Cs=inf  Measurements=on
  IGBT AYN2 : spsIGBTLib/IGBT  Ron=0.001  Lon=0  Vf=1  Tf=1e-6  Tt=2e-6  IC=0  Rs=1e5  Cs=inf  Measurements=on
  IGBT AYP2 : spsIGBTLib/IGBT  Ron=0.001  Lon=0  Vf=1  Tf=1e-6  Tt=2e-6  IC=0  Rs=1e5  Cs=inf  Measurements=on
  IGBT BDN2 : spsIGBTLib/IGBT  Ron=0.001  Lon=0  Vf=1  Tf=1e-6  Tt=2e-6  IC=0  Rs=1e5  Cs=inf  Measurements=on
  IGBT BDP2 : spsIGBTLib/IGBT  Ron=0.001  Lon=0  Vf=1  Tf=1e-6  Tt=2e-6  IC=0  Rs=1e5  Cs=inf  Measurements=on
  IGBT BYN2 : spsIGBTLib/IGBT  Ron=0.001  Lon=0  Vf=1  Tf=1e-6  Tt=2e-6  IC=0  Rs=1e5  Cs=inf  Measurements=on
  IGBT BYP2 : spsIGBTLib/IGBT  Ron=0.001  Lon=0  Vf=1  Tf=1e-6  Tt=2e-6  IC=0  Rs=1e5  Cs=inf  Measurements=on
  IGBT CDN2 : spsIGBTLib/IGBT  Ron=0.001  Lon=0  Vf=1  Tf=1e-6  Tt=2e-6  IC=0  Rs=1e5  Cs=inf  Measurements=on
  IGBT CDP2 : spsIGBTLib/IGBT  Ron=0.001  Lon=0  Vf=1  Tf=1e-6  Tt=2e-6  IC=0  Rs=1e5  Cs=inf  Measurements=on
  IGBT CYN2 : spsIGBTLib/IGBT  Ron=0.001  Lon=0  Vf=1  Tf=1e-6  Tt=2e-6  IC=0  Rs=1e5  Cs=inf  Measurements=on
  IGBT CYP2 : spsIGBTLib/IGBT  Ron=0.001  Lon=0  Vf=1  Tf=1e-6  Tt=2e-6  IC=0  Rs=1e5  Cs=inf  Measurements=on
  Series RLC Branch : spsSeriesRLCBranchLib/Series RLC Branch  LConnTagsString=__new0  RConnTagsString=__new0  BranchType=L  Resistance=1  Inductance=0.0004  SetiL0=off  InitialCurrent=0  Capacitance=1e-6  Setx0=off  InitialVoltage=0  Measurements=None
  Series RLC Branch1 : spsSeriesRLCBranchLib/Series RLC Branch  LConnTagsString=__new0  RConnTagsString=__new0  BranchType=L  Resistance=1  Inductance=0.0004  SetiL0=off  InitialCurrent=0  Capacitance=1e-6  Setx0=off  InitialVoltage=0  Measurements=None
  Series RLC Branch{2..7} (6 alike) : spsSeriesRLCBranchLib/Series RLC Branch  LConnTagsString=__new0  RConnTagsString=__new0  BranchType=RL  Resistance=R_12_arm  Inductance=1e-3  SetiL0=off  InitialCurrent=0  Capacitance=1e-6  Setx0=off  InitialVoltage=0  Measurements=None
  Terminator{,1..11} (12 alike) : Terminator
  Three-Phase V-I Measurement : spsThreePhaseVIMeasurementLib/Three-Phase V-I Measurement  VoltageMeasurement=phase-to-ground  SetLabelV=off  LabelV=Vabc  Vpu=off  VpuLL=off  CurrentMeasurement=yes  SetLabelI=off  LabelI=Iabc  Ipu=off  Pbase=100e6  Vbase=500e3  OutputType=Complex  PhasorSimulation=off  PSBequivalent=0
  Tr3 : spsThreePhaseTransformerThreeWindingsLib/Three-Phase Transformer (Three Windings)  Winding1Connection=Yg  Winding2Connection=Y  Winding3Connection=Delta (D1)  CoreType=Three single-phase transformers  SetSaturation=off  Hysteresis=off  DataFile='hysteresis'  SetInitialFlux=off  Measurements=None  UNITS=pu  NominalPower=[ 2.5e9 , 60 ]  Winding1=[ 4e+5 *0.1, 0.002 , 0.08 ]  Winding2=[ 2.675e+5 , 0.002 , 0.08 ]  Winding3=[ 2.675e+5 , 0.002 , 0.08 ]  Rm=1000  Lm=1000  L0=0.5  Saturation=[ 0,0 ; 0.0024,1.2 ; 1.0,1.52 ]  InitialFluxes=[0.8 -0.8 0.7]  BreakLoop=off  DiscreteSolver=Trapezoidal iterative  DataType=off  TransfoNumber=1
      settings: LibrarySourceBlock=|
      | sps_lib/Power Grid Elements/Three-Phase
      | Transformer
      | (Three Windings)
  Voltage Measurement : spsVoltageMeasurementLib/Voltage Measurement  PhasorSimulation=off  OutputType=Complex  PSBequivalent=0
  Voltage Measurement1 : spsVoltageMeasurementLib/Voltage Measurement  PhasorSimulation=off  OutputType=Complex  PSBequivalent=0
  Voltage Measurement2 : spsVoltageMeasurementLib/Voltage Measurement  PhasorSimulation=off  OutputType=Complex  PSBequivalent=0
  A : PMIOPort  Side=Left
  B : PMIOPort  Port=2  Side=Left
  C : PMIOPort  Port=3  Side=Left
  P : PMIOPort  Port=4  Side=Right
  N : PMIOPort  Port=5  Side=Right
  tag scope: Isec3=global, V_D2=global, V_Y2=global, V_rectifier2=global, Vsec3=global
  wires:
  IGBT AYN2/1 -> Terminator3/1
  [ADN2] -> IGBT ADN2/1
  [AYP2] -> IGBT AYP2/1
  [BDN2] -> IGBT BDN2/1
  [CYN2] -> IGBT CYN2/1
  [CDP2] -> IGBT CDP2/1
  [ADP2] -> IGBT ADP2/1
  IGBT CDN2/1 -> Terminator11/1
  IGBT BYN2/1 -> Terminator4/1
  [AYN2] -> IGBT AYN2/1
  [CYP2] -> IGBT CYP2/1
  [BYP2] -> IGBT BYP2/1
  IGBT CYN2/1 -> Terminator5/1
  IGBT BDN2/1 -> Terminator10/1
  IGBT ADP2/1 -> Terminator6/1
  [CDN2] -> IGBT CDN2/1
  IGBT ADN2/1 -> Terminator9/1
  IGBT AYP2/1 -> Terminator/1
  [BYN2] -> IGBT BYN2/1
  [BDP2] -> IGBT BDP2/1
  IGBT CDP2/1 -> Terminator8/1
  IGBT BDP2/1 -> Terminator7/1
  IGBT BYP2/1 -> Terminator1/1
  IGBT CYP2/1 -> Terminator2/1
  Voltage Measurement/1 -> [V_Y2]
  Voltage Measurement1/1 -> [V_D2]
  Three-Phase V-I Measurement/1 -> [Vsec3]
  Three-Phase V-I Measurement/2 -> [Isec3]
  Voltage Measurement2/1 -> [V_rectifier2]
  connections:
  IGBT BDN2/RConn1 -- Series RLC Branch6/RConn1 -- IGBT BDP2/LConn1
  IGBT AYN2/LConn1 -- Voltage Measurement1/LConn1 -- Voltage Measurement/LConn2 -- IGBT BDP2/RConn1 -- IGBT CDP2/RConn1 -- IGBT ADP2/RConn1 -- IGBT CYN2/LConn1 -- IGBT BYN2/LConn1
  IGBT AYP2/RConn1 -- IGBT BYP2/RConn1 -- Series RLC Branch/LConn1 -- Voltage Measurement/LConn1 -- IGBT CYP2/RConn1
  IGBT AYN2/RConn1 -- Series RLC Branch2/LConn1 -- IGBT AYP2/LConn1
  IGBT CYN2/RConn1 -- Series RLC Branch4/LConn1 -- IGBT CYP2/LConn1
  IGBT BYN2/RConn1 -- Series RLC Branch3/LConn1 -- IGBT BYP2/LConn1
  IGBT ADN2/RConn1 -- Series RLC Branch7/RConn1 -- IGBT ADP2/LConn1
  IGBT CDN2/RConn1 -- Series RLC Branch5/RConn1 -- IGBT CDP2/LConn1
  IGBT ADN2/LConn1 -- IGBT BDN2/LConn1 -- Series RLC Branch1/LConn1 -- Voltage Measurement1/LConn2 -- IGBT CDN2/LConn1
  Tr3/LConn1 -- Three-Phase V-I Measurement/RConn1
  Tr3/LConn3 -- Three-Phase V-I Measurement/RConn3
  Tr3/LConn2 -- Three-Phase V-I Measurement/RConn2
  A/RConn1 -- Three-Phase V-I Measurement/LConn1
  B/RConn1 -- Three-Phase V-I Measurement/LConn2
  C/RConn1 -- Three-Phase V-I Measurement/LConn3
  C_rectifier2/LConn1 -- P/RConn1 -- Voltage Measurement2/LConn1 -- Series RLC Branch/RConn1
  N/RConn1 -- Series RLC Branch1/RConn1 -- C_rectifier2/RConn1 -- Voltage Measurement2/LConn2
  Tr3/RConn1 -- Series RLC Branch2/RConn1
  Tr3/RConn2 -- Series RLC Branch3/RConn1
  Tr3/RConn3 -- Series RLC Branch4/RConn1
  Tr3/RConn5 -- Series RLC Branch6/LConn1
  Tr3/RConn4 -- Series RLC Branch7/LConn1
  Tr3/RConn6 -- Series RLC Branch5/LConn1

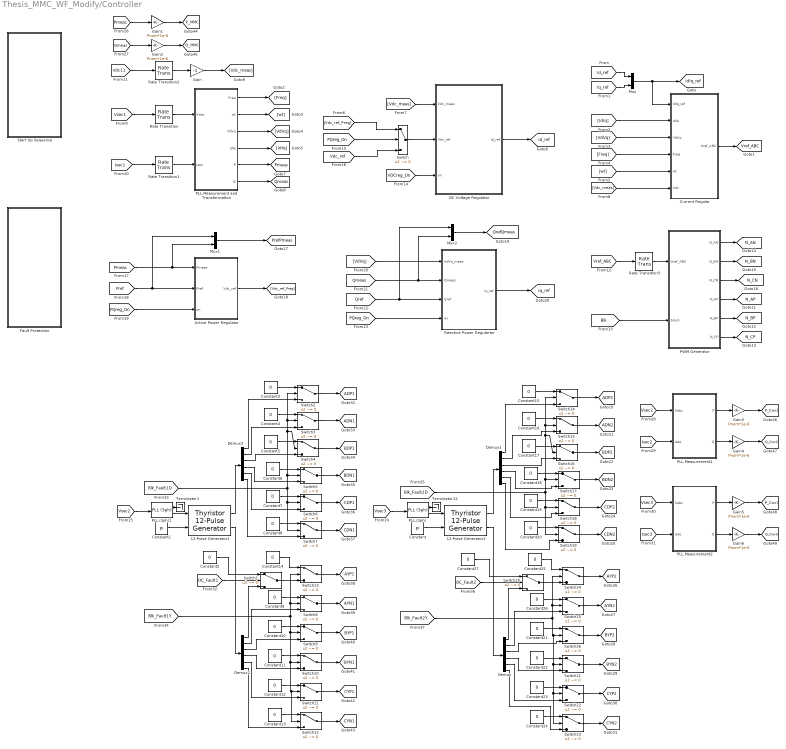
== system Thesis_MMC_WF_Modify/Controller ==
  12-Pulse Generator1 : eeThyristorTwelvePulseGenerator/Thyristor 12-Pulse Generator  Ord=Sequential device order  Dcon=Lagging (Delta1)  Pw=5*pi/6  Ts=Ts_Control
      settings: LibrarySourceBlock=|
      | ee_sl_lib/Pulse Width
      | Modulation/Thyristor 12-Pulse
      | Generator
  12-Pulse Generator2 : eeThyristorTwelvePulseGenerator/Thyristor 12-Pulse Generator  Ord=Sequential device order  Dcon=Lagging (Delta1)  Pw=5*pi/6  Ts=Ts_Control
      settings: LibrarySourceBlock=|
      | ee_sl_lib/Pulse Width
      | Modulation/Thyristor 12-Pulse
      | Generator
  Active Power Regulator : Subsystem
  Constant : Constant  Value=pi
  Constant1 : Constant  Value=pi
  Constant{2..27} (26 alike) : Constant  Value=0
  Current Regular : Subsystem
  DC Voltage Regulator : Subsystem
  Demux{,1..3} (4 alike) : Demux  Outputs=6
  Fault Protection : Subsystem
  Gain : Gain  Gain=-1
  Gain{1..6} (6 alike) : Gain  Gain=Pnom*1e-6
  Mux : Mux  Inputs=2
  Mux1 : Mux  Inputs=2
  Mux2 : Mux  Inputs=2
  PLL (3ph) : spsPLL3phLib/PLL (3ph)  Fmin=45  Par_Init=[0, 60]  ParK=[180, 3200, 1]  TcD=1e-4  MaxRateChangeFreq=12  FilterCutOffFreq=25  Ts=Ts_Control  AGC=on
  PLL (3ph)1 : spsPLL3phLib/PLL (3ph)  Fmin=45  Par_Init=[0, 60]  ParK=[180, 3200, 1]  TcD=1e-4  MaxRateChangeFreq=12  FilterCutOffFreq=25  Ts=Ts_Control  AGC=on
  PLL,Measurement and Transformation : Subsystem
  PLL,Measurement1 : Subsystem
  PLL,Measurement2 : Subsystem
  PWM Generator : Subsystem
  Rate Transition : RateTransition  OutPortSampleTime=Ts_Control
  Rate Transition1 : RateTransition  OutPortSampleTime=Ts_Control
  Rate Transition2 : RateTransition  OutPortSampleTime=Ts_Control
  Rate Transition3 : RateTransition  OutPortSampleTime=Ts_Power
  Reactive Power Regulartor : Subsystem
  Start Up Sequence : Subsystem
  Switch{,1..26} (27 alike) : Switch  Criteria=u2 ~= 0  SaturateOnIntegerOverflow=off  InputSameDT=off
  Terminator1 : Terminator
  Terminator12 : Terminator
  tag scope: ADN1=global, ADN2=global, ADP1=global, ADP2=global, AYN1=global, AYN2=global, AYP1=global, AYP2=global, BDN1=global, BDN2=global, BDP1=global, BDP2=global, BYN1=global, BYN2=global, BYP1=global, BYP2=global, CDN1=global, CDN2=global, CDP1=global, CDP2=global, CYN1=global, CYN2=global, CYP1=global, CYP2=global, IdIq_ref=global, Id_ref=global, Iq_ref=global, N_AN=global, N_AP=global, N_BN=global, N_BP=global, N_CN=global, N_CP=global, P_Cov2=global, P_Cov3=global, P_MMC=global, Pmeas=global, PrefPmeas=global, Q_Cov2=global, Q_Cov3=global, Q_MMC=global, Qmeas=global, QrefQmeas=global, Vref_ABC=global
  wires:
  DC Voltage Regulator/1(Id_ref) -> [Id_ref]
  [Id_ref] -> Mux/1
  [Iq_ref] -> Mux/2
  Mux/1 -> Current Regular/1(IdIq_ref), [IdIq_ref]
  [IdIq] -> Current Regular/2(IdIq)
  [VdVq] -> Current Regular/3(VdVq)
  [Freq] -> Current Regular/4(Freq)
  [wt] -> Current Regular/5(wt)
  [Vdc_meas] -> Current Regular/6(Vdc)
  Current Regular/1(Uref_ABC) -> [Vref_ABC]
  [Vsec1] -> Rate Transition/1
  Rate Transition/1 -> PLL,Measurement and Transformation/1(Vabc)
  [Isec1] -> Rate Transition1/1
  Rate Transition1/1 -> PLL,Measurement and Transformation/2(Iabc)
  PLL,Measurement and Transformation/1(Freq) -> [Freq]
  PLL,Measurement and Transformation/2(wt) -> [wt]
  PLL,Measurement and Transformation/3(VdVq) -> [VdVq]
  PLL,Measurement and Transformation/4(IdIq) -> [IdIq]
  PLL,Measurement and Transformation/5(P) -> [Pmeas]
  PLL,Measurement and Transformation/6(Q) -> [Qmeas]
  [Vdc11] -> Rate Transition2/1
  [Vref_ABC] -> Rate Transition3/1
  Rate Transition3/1 -> PWM Generator/1(Uref_ABC)
  [Blk] -> PWM Generator/2(block)
  [Vdc_meas] -> DC Voltage Regulator/1(Vdc_meas)
  [VDCreg_On] -> DC Voltage Regulator/3(on)
  [PQreg_On] -> Switch/2
  [PQreg_On] -> Active Power Regulator/3(on)
  [Pref] -> Mux1/1, Active Power Regulator/2(Pref)
  [Pmeas] -> Active Power Regulator/1(Pmeas), Mux1/2
  Mux1/1 -> [PrefPmeas]
  Active Power Regulator/1(Vdc_ref) -> [Vdc_ref_Preg]
  [VdVq] -> Reactive Power Regulartor/1(VdVq_meas)
  [Qmeas] -> Mux2/2, Reactive Power Regulartor/2(Qmeas)
  [Qref] -> Mux2/1, Reactive Power Regulartor/3(Qref)
  [PQreg_On] -> Reactive Power Regulartor/4(on)
  Mux2/1 -> [QrefQmeas]
  Reactive Power Regulartor/1(Iq_ref) -> [Iq_ref]
  [Vdc_ref_Preg] -> Switch/1
  [Vdc_ref] -> Switch/3
  Switch/1 -> DC Voltage Regulator/2(Vdc_ref)
  PWM Generator/4(N_AP) -> [N_AP]
  PWM Generator/1(N_AN) -> [N_AN]
  PWM Generator/5(N_BP) -> [N_BP]
  PWM Generator/2(N_BN) -> [N_BN]
  PWM Generator/3(N_CN) -> [N_CN]
  PWM Generator/6(N_CP) -> [N_CP]
  [Vsec3] -> PLL (3ph)/1
  12-Pulse Generator2/1 -> Demux1/1
  PLL (3ph)/2 -> 12-Pulse Generator2/1
  PLL (3ph)/1 -> Terminator12/1
  Constant/1 -> 12-Pulse Generator2/2
  12-Pulse Generator2/2 -> Demux/1
  12-Pulse Generator1/2 -> Demux2/1
  PLL (3ph)1/1 -> Terminator1/1
  Constant1/1 -> 12-Pulse Generator1/2
  12-Pulse Generator1/1 -> Demux3/1
  [Vsec2] -> PLL (3ph)1/1
  PLL (3ph)1/2 -> 12-Pulse Generator1/1
  Gain2/1 -> [Q_MMC]
  [Pmeas] -> Gain1/1
  Gain1/1 -> [P_MMC]
  [Qmeas] -> Gain2/1
  Rate Transition2/1 -> Gain/1
  Gain/1 -> [Vdc_meas]
  [Vsec3] -> PLL,Measurement2/1(Vabc)
  [Isec3] -> PLL,Measurement2/2(Iabc)
  [Isec2] -> PLL,Measurement1/2(Iabc)
  [Vsec2] -> PLL,Measurement1/1(Vabc)
  PLL,Measurement2/2(Q) -> Gain6/1
  Gain3/1 -> [P_Cov2]
  Gain4/1 -> [Q_Cov2]
  PLL,Measurement1/2(Q) -> Gain4/1
  Demux2/1 -> Switch1/3
  [OC_Fault1] -> Switch1/2
  Constant2/1 -> Switch1/1
  PLL,Measurement1/1(P) -> Gain3/1
  PLL,Measurement2/1(P) -> Gain5/1
  Gain5/1 -> [P_Cov3]
  Gain6/1 -> [Q_Cov3]
  Constant3/1 -> Switch2/1
  Switch2/1 -> [ADP1]
  Constant4/1 -> Switch3/1
  Switch3/1 -> [ADN1]
  Demux3/1 -> Switch2/3
  Demux3/2 -> Switch3/3
  Constant5/1 -> Switch4/1
  Switch4/1 -> [BDP1]
  Constant6/1 -> Switch5/1
  Switch5/1 -> [BDN1]
  Constant7/1 -> Switch6/1
  Switch6/1 -> [CDP1]
  Constant8/1 -> Switch7/1
  Switch7/1 -> [CDN1]
  Demux3/3 -> Switch4/3
  Demux3/4 -> Switch5/3
  Demux3/5 -> Switch6/3
  Demux3/6 -> Switch7/3
  Constant9/1 -> Switch8/1
  Switch8/1 -> [AYN1]
  Constant10/1 -> Switch9/1
  Switch9/1 -> [BYP1]
  Constant11/1 -> Switch10/1
  Switch10/1 -> [BYN1]
  Constant12/1 -> Switch11/1
  Switch11/1 -> [CYP1]
  Constant13/1 -> Switch12/1
  Switch12/1 -> [CYN1]
  Demux2/2 -> Switch8/3
  Demux2/3 -> Switch9/3
  Demux2/4 -> Switch10/3
  Demux2/5 -> Switch11/3
  Demux2/6 -> Switch12/3
  Switch1/1 -> Switch13/3
  Switch13/1 -> [AYP1]
  Constant14/1 -> Switch13/1
  [Blk_Fault1D] -> Switch2/2, Switch3/2, Switch4/2, Switch5/2, Switch7/2, Switch6/2
  [Blk_Fault1Y] -> Switch8/2, Switch13/2, Switch12/2, Switch11/2, Switch10/2, Switch9/2
  Switch19/1 -> [CDN2]
  Demux1/2 -> Switch15/3
  Demux1/4 -> Switch17/3
  Constant18/1 -> Switch17/1
  Constant16/1 -> Switch15/1
  Switch14/1 -> [ADP2]
  Switch16/1 -> [BDP2]
  Demux1/6 -> Switch19/3
  Switch15/1 -> [ADN2]
  Constant19/1 -> Switch18/1
  Constant15/1 -> Switch14/1
  Demux1/5 -> Switch18/3
  Constant17/1 -> Switch16/1
  Demux1/3 -> Switch16/3
  Demux1/1 -> Switch14/3
  Switch17/1 -> [BDN2]
  Constant20/1 -> Switch19/1
  Switch18/1 -> [CDP2]
  [Blk_Fault2D] -> Switch14/2, Switch15/2, Switch16/2, Switch17/2, Switch19/2, Switch18/2
  Constant26/1 -> Switch25/1
  Demux/5 -> Switch22/3
  Constant24/1 -> Switch23/1
  Switch22/1 -> [CYP2]
  Demux/3 -> Switch26/3
  Demux/4 -> Switch21/3
  Constant21/1 -> Switch26/1
  Demux/6 -> Switch23/3
  Switch23/1 -> [CYN2]
  Constant22/1 -> Switch21/1
  Switch24/1 -> [AYP2]
  Switch20/1 -> Switch24/3
  Constant27/1 -> Switch20/1
  Demux/1 -> Switch20/3
  Switch26/1 -> [BYP2]
  [OC_Fault2] -> Switch20/2
  Demux/2 -> Switch25/3
  Constant25/1 -> Switch24/1
  [Blk_Fault2Y] -> Switch25/2, Switch24/2, Switch23/2, Switch22/2, Switch21/2, Switch26/2
  Switch21/1 -> [BYN2]
  Constant23/1 -> Switch22/1
  Switch25/1 -> [AYN2]

== system Thesis_MMC_WF_Modify/Farm1 ==
  Three-Phase V-I Measurement : spsThreePhaseVIMeasurementLib/Three-Phase V-I Measurement  VoltageMeasurement=phase-to-ground  SetLabelV=off  LabelV=Vabc  Vpu=off  VpuLL=off  CurrentMeasurement=yes  SetLabelI=off  LabelI=Iabc  Ipu=off  Pbase=100e6  Vbase=500e3  OutputType=Complex  PhasorSimulation=off  PSBequivalent=0
  A : PMIOPort  Side=Left
  B : PMIOPort  Port=2  Side=Left
  a : PMIOPort  Port=3  Side=Right
  b : PMIOPort  Port=4  Side=Right
  C : PMIOPort  Port=5  Side=Left
  c : PMIOPort  Port=6  Side=Right
  tag scope: IFarm1=global, VFarm1=global
  wires:
  Three-Phase V-I Measurement/2 -> [IFarm1]
  Three-Phase V-I Measurement/1 -> [VFarm1]
  connections:
  Three-Phase V-I Measurement/LConn1 -- A/RConn1
  Three-Phase V-I Measurement/RConn2 -- b/RConn1
  Three-Phase V-I Measurement/LConn2 -- B/RConn1
  Three-Phase V-I Measurement/RConn3 -- c/RConn1
  Three-Phase V-I Measurement/RConn1 -- a/RConn1
  Three-Phase V-I Measurement/LConn3 -- C/RConn1

== system Thesis_MMC_WF_Modify/Farm2 ==
  Three-Phase V-I Measurement : spsThreePhaseVIMeasurementLib/Three-Phase V-I Measurement  VoltageMeasurement=phase-to-ground  SetLabelV=off  LabelV=Vabc  Vpu=off  VpuLL=off  CurrentMeasurement=yes  SetLabelI=off  LabelI=Iabc  Ipu=off  Pbase=100e6  Vbase=500e3  OutputType=Complex  PhasorSimulation=off  PSBequivalent=0
  A : PMIOPort  Side=Left
  B : PMIOPort  Port=2  Side=Left
  a : PMIOPort  Port=3  Side=Right
  b : PMIOPort  Port=4  Side=Right
  C : PMIOPort  Port=5  Side=Left
  c : PMIOPort  Port=6  Side=Right
  tag scope: IFarm2=global, VFarm2=global
  wires:
  Three-Phase V-I Measurement/2 -> [IFarm2]
  Three-Phase V-I Measurement/1 -> [VFarm2]
  connections:
  Three-Phase V-I Measurement/LConn1 -- A/RConn1
  Three-Phase V-I Measurement/RConn2 -- b/RConn1
  Three-Phase V-I Measurement/LConn2 -- B/RConn1
  Three-Phase V-I Measurement/RConn3 -- c/RConn1
  Three-Phase V-I Measurement/RConn1 -- a/RConn1
  Three-Phase V-I Measurement/LConn3 -- C/RConn1

== system Thesis_MMC_WF_Modify/Farm3 ==
  Three-Phase V-I Measurement : spsThreePhaseVIMeasurementLib/Three-Phase V-I Measurement  VoltageMeasurement=phase-to-ground  SetLabelV=off  LabelV=Vabc  Vpu=off  VpuLL=off  CurrentMeasurement=yes  SetLabelI=off  LabelI=Iabc  Ipu=off  Pbase=100e6  Vbase=500e3  OutputType=Complex  PhasorSimulation=off  PSBequivalent=0
  A : PMIOPort  Side=Left
  B : PMIOPort  Port=2  Side=Left
  a : PMIOPort  Port=3  Side=Right
  b : PMIOPort  Port=4  Side=Right
  C : PMIOPort  Port=5  Side=Left
  c : PMIOPort  Port=6  Side=Right
  tag scope: IFarm3=global, VFarm3=global
  wires:
  Three-Phase V-I Measurement/2 -> [IFarm3]
  Three-Phase V-I Measurement/1 -> [VFarm3]
  connections:
  Three-Phase V-I Measurement/LConn1 -- A/RConn1
  Three-Phase V-I Measurement/RConn2 -- b/RConn1
  Three-Phase V-I Measurement/LConn2 -- B/RConn1
  Three-Phase V-I Measurement/RConn3 -- c/RConn1
  Three-Phase V-I Measurement/RConn1 -- a/RConn1
  Three-Phase V-I Measurement/LConn3 -- C/RConn1

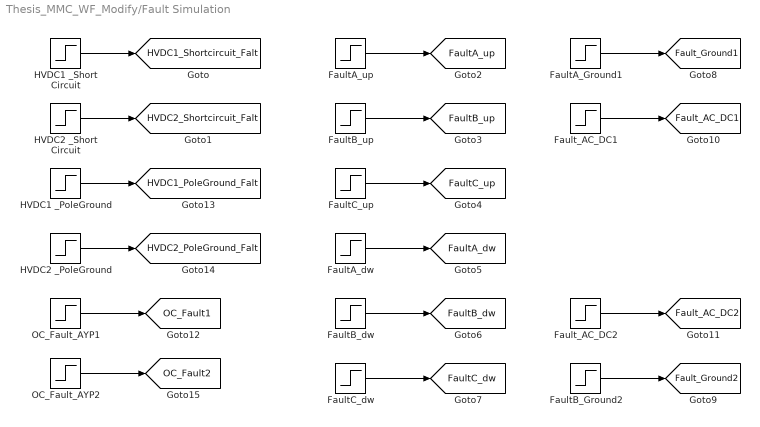
== system Thesis_MMC_WF_Modify/Fault Simulation ==
  FaultA_Ground1 : Step  Time=99999  SampleTime=0
  FaultA_dw : Step  Time=9999999  SampleTime=0
  FaultA_up : Step  Time=999999  SampleTime=0
  FaultB_Ground2 : Step  Time=9999999  SampleTime=0
  FaultB_dw : Step  Time=999999  SampleTime=0
  FaultB_up : Step  Time=99999  SampleTime=0
  FaultC_dw : Step  Time=9999999  SampleTime=0
  FaultC_up : Step  Time=999999  SampleTime=0
  Fault_AC_DC1 : Step  Time=999999  SampleTime=0
  Fault_AC_DC2 : Step  Time=9999999  SampleTime=0
  HVDC1 _PoleGround : Step  Time=99999  SampleTime=0
  HVDC1 _Short Circuit : Step  Time=999999  SampleTime=0
  HVDC2 _PoleGround : Step  Time=99999  SampleTime=0
  HVDC2 _Short Circuit : Step  Time=99999  SampleTime=0
  OC_Fault_AYP1 : Step  Time=T_Fault  SampleTime=0
  OC_Fault_AYP2 : Step  Time=999999  SampleTime=0
  tag scope: FaultA_dw=global, FaultA_up=global, FaultB_dw=global, FaultB_up=global, FaultC_dw=global, FaultC_up=global, Fault_AC_DC1=global, Fault_AC_DC2=global, Fault_Ground1=global, Fault_Ground2=global, HVDC1_PoleGround_Falt=global, HVDC1_Shortcircuit_Falt=global, HVDC2_PoleGround_Falt=global, HVDC2_Shortcircuit_Falt=global, OC_Fault1=global, OC_Fault2=global
  wires:
  HVDC1 _Short Circuit/1 -> [HVDC1_Shortcircuit_Falt]
  HVDC2 _Short Circuit/1 -> [HVDC2_Shortcircuit_Falt]
  FaultB_up/1 -> [FaultB_up]
  FaultA_up/1 -> [FaultA_up]
  FaultA_dw/1 -> [FaultA_dw]
  FaultC_up/1 -> [FaultC_up]
  FaultC_dw/1 -> [FaultC_dw]
  FaultB_dw/1 -> [FaultB_dw]
  FaultB_Ground2/1 -> [Fault_Ground2]
  FaultA_Ground1/1 -> [Fault_Ground1]
  Fault_AC_DC2/1 -> [Fault_AC_DC2]
  Fault_AC_DC1/1 -> [Fault_AC_DC1]
  OC_Fault_AYP1/1 -> [OC_Fault1]
  HVDC2 _PoleGround/1 -> [HVDC2_PoleGround_Falt]
  HVDC1 _PoleGround/1 -> [HVDC1_PoleGround_Falt]
  OC_Fault_AYP2/1 -> [OC_Fault2]

== system Thesis_MMC_WF_Modify/HVDC Line1 ==
  Constant : Constant  Value=1e-6
  Current Measurement : spsCurrentMeasurementLib/Current Measurement  PhasorSimulation=off  OutputType=Complex  PSBequivalent=0
  Fault1 : spsIdealSwitchLib/Ideal Switch  Ron=1  Lon=0  IC=0  Rs=1e6  Cs=inf  Measurements=off
  Fault2 : spsIdealSwitchLib/Ideal Switch  Ron=1  Lon=0  IC=0  Rs=1e6  Cs=inf  Measurements=off
  Ground : spsGroundLib/Ground  LConnTagsString=a
  Product : Product  Inputs=3
  Series RLC Branch{1..4} (4 alike) : spsSeriesRLCBranchLib/Series RLC Branch  LConnTagsString=__new0  RConnTagsString=__new0  BranchType=RL  Resistance=R_cable/2  Inductance=L_cable/2  SetiL0=off  InitialCurrent=0  Capacitance=1e-6  Setx0=off  InitialVoltage=0  Measurements=None
  Voltage Measurement : spsVoltageMeasurementLib/Voltage Measurement  PhasorSimulation=off  OutputType=Complex  PSBequivalent=0
  1 : PMIOPort  Side=Left
  2 : PMIOPort  Port=2  Side=Left
  Conn1 : PMIOPort  Port=3  Side=Right
  Conn2 : PMIOPort  Port=4  Side=Right
  tag scope: Idc1=global, P_HVDC1=global, Vdc1=global
  wires:
  Current Measurement/1 -> [Idc1]
  Voltage Measurement/1 -> [Vdc1]
  [HVDC1_Shortcircuit_Falt] -> Fault1/1
  [HVDC1_Shortcircuit_Falt] -> Fault2/1
  [Idc1] -> Product/1
  [Vdc1] -> Product/2
  Product/1 -> [P_HVDC1]
  Constant/1 -> Product/3
  connections:
  Series RLC Branch2/LConn1 -- Fault2/LConn1 -- Fault1/LConn1 -- Series RLC Branch1/RConn1
  Series RLC Branch4/RConn1 -- Conn2/RConn1
  Series RLC Branch4/LConn1 -- Fault1/RConn1 -- Series RLC Branch3/RConn1
  Series RLC Branch3/LConn1 -- Voltage Measurement/LConn2 -- 2/RConn1
  Series RLC Branch2/RConn1 -- Conn1/RConn1
  1/RConn1 -- Voltage Measurement/LConn1 -- Current Measurement/LConn1
  Current Measurement/RConn1 -- Series RLC Branch1/LConn1
  Ground/LConn1 -- Fault2/RConn1

== system Thesis_MMC_WF_Modify/HVDC Line2 ==
  Constant : Constant  Value=1e-6
  Current Measurement : spsCurrentMeasurementLib/Current Measurement  PhasorSimulation=off  OutputType=Complex  PSBequivalent=0
  Fault1 : spsIdealSwitchLib/Ideal Switch  Ron=1  Lon=0  IC=0  Rs=1e6  Cs=inf  Measurements=off
  Fault2 : spsIdealSwitchLib/Ideal Switch  Ron=1  Lon=0  IC=0  Rs=1e6  Cs=inf  Measurements=off
  Ground : spsGroundLib/Ground  LConnTagsString=a
  Product : Product  Inputs=3
  Series RLC Branch{1..4} (4 alike) : spsSeriesRLCBranchLib/Series RLC Branch  LConnTagsString=__new0  RConnTagsString=__new0  BranchType=RL  Resistance=R_cable/2  Inductance=L_cable/2  SetiL0=off  InitialCurrent=0  Capacitance=1e-6  Setx0=off  InitialVoltage=0  Measurements=None
  Voltage Measurement : spsVoltageMeasurementLib/Voltage Measurement  PhasorSimulation=off  OutputType=Complex  PSBequivalent=0
  1 : PMIOPort  Side=Left
  2 : PMIOPort  Port=2  Side=Left
  Conn1 : PMIOPort  Port=3  Side=Right
  Conn2 : PMIOPort  Port=4  Side=Right
  tag scope: Idc3=global, P_HVDC2=global, Vdc3=global
  wires:
  Current Measurement/1 -> [Idc3]
  Voltage Measurement/1 -> [Vdc3]
  [HVDC2_Shortcircuit_Falt] -> Fault1/1
  [HVDC2_PoleGround_Falt] -> Fault2/1
  [Vdc3] -> Product/2
  [Idc3] -> Product/1
  Product/1 -> [P_HVDC2]
  Constant/1 -> Product/3
  connections:
  Series RLC Branch2/LConn1 -- Fault1/LConn1 -- Series RLC Branch1/RConn1 -- Fault2/LConn1
  Series RLC Branch4/RConn1 -- Conn2/RConn1
  Series RLC Branch4/LConn1 -- Fault1/RConn1 -- Series RLC Branch3/RConn1
  Series RLC Branch3/LConn1 -- Voltage Measurement/LConn2 -- 2/RConn1
  Series RLC Branch2/RConn1 -- Conn1/RConn1
  1/RConn1 -- Voltage Measurement/LConn1 -- Current Measurement/LConn1
  Current Measurement/RConn1 -- Series RLC Branch1/LConn1
  Ground/LConn1 -- Fault2/RConn1
